simulink model "LAB_2_A3"  (R2021b)
settings: Solver=FixedStepAuto  StartTime=0.0  StopTime=20  FixedStep=0.05  RelTol=1e-3
settings Model: Creator=rfv84  LastModifiedBy=rfv84
settings DataIOCC: SaveOutput=off  SignalLogging=off  DSMLogging=off  SaveTime=off  ReturnWorkspaceOutputs=off

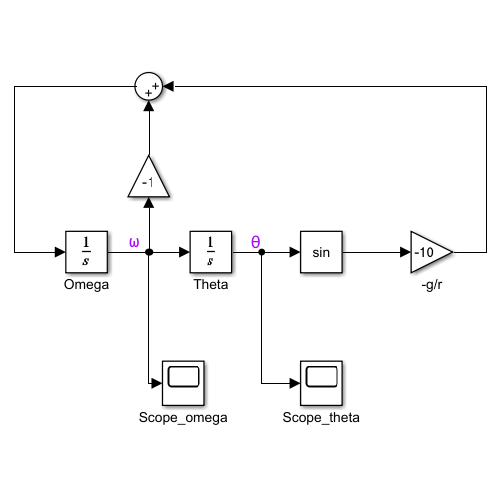
[thumbnail: Simulink's stored preview of the top-level diagram]
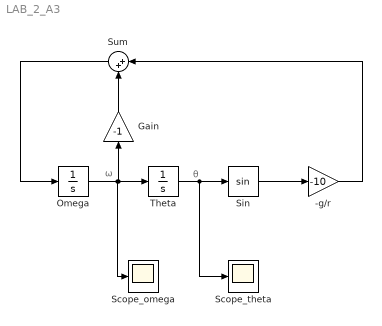
== system LAB_2_A3 ==
  note: ω
  note: θ
  -g/r : Gain  Gain=-10
  Gain : Gain  Gain=-1
  Omega : Integrator  InitialCondition=-2
  Scope_omega : Scope
  Scope_theta : Scope
  Sin : Trigonometry
  Sum : Sum  Inputs=|++
  Theta : Integrator  InitialCondition=3
  wires:
  Omega/1 -> Gain/1, Theta/1, Scope_omega/1
  Theta/1 -> Scope_theta/1, Sin/1
  Sin/1 -> -g/r/1
  Gain/1 -> Sum/2
  -g/r/1 -> Sum/1
  Sum/1 -> Omega/1
